simulink model "ACC_RL_new"  (R2022a)
settings: Solver=FixedStepAuto  StartTime=0.0  StopTime=T  FixedStep=Ts  RelTol=1e-3
StartFcn:
  | a_lead_seed = simCount;
  | simCount = simCount + 1;
undefined symbols (not defined in the file): amax_ego, amax_lead, amin_ego, amin_lead, change_freq, D_default, isTerminate, rewardWeights, t_gap, Ts, v0_ego, v0_lead, v_set, x0_ego, x0_lead
libraries: simulink x5, rllib x1
settings Model: Creator=The MathWorks, Inc.  LastModifiedBy=momentumlab
settings SolverCC: AlgebraicLoopSolver=TrustRegion
settings DataIOCC: ReturnWorkspaceOutputs=off
settings DebuggingCC: UnconnectedInputMsg=warning  UnconnectedOutputMsg=warning  UnconnectedLineMsg=warning  SFMachineParentedDataDiag=warning  ArithmeticOperatorsInVariantConditions=warning
settings SFSimCC: SimUseLocalCustomCode=off  CustomCodeUndefinedFunction=UseInterfaceOnly
settings RTWCC: RTWUseLocalCustomCode=off  DLArmComputeVersion=19.05
settings CodeAppCC: StateflowObjectComments=on

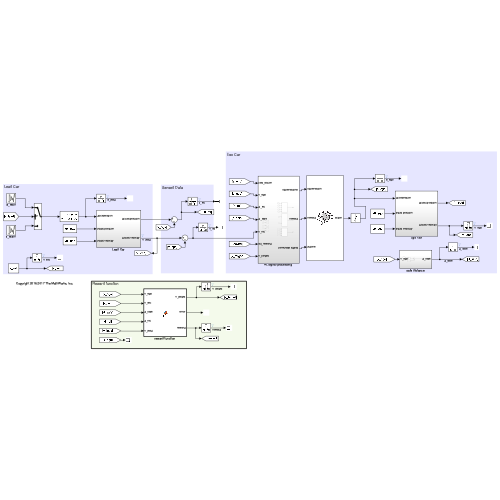
[thumbnail: Simulink's stored preview of the top-level diagram]
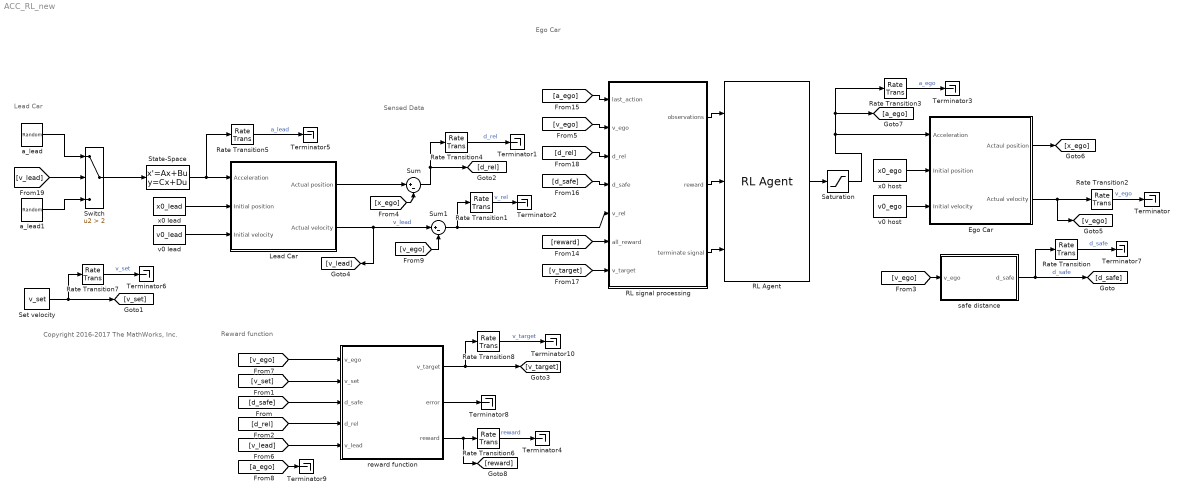
== system ACC_RL_new ==
  note: Reward function
  note: Sensed Data
  note: Lead Car
  note: Ego Car
  note: Copyright 2016-2017 The MathWorks, Inc.
  Ego Car : Subsystem
  Lead Car : Subsystem
  RL Agent : rllib/RL Agent  Agent=agent  ExternalActionAsInput=off  ProvideLastAction=off  ProvideCumRwd=off  TreatAsDirectFeedthrough=on  UseStrictObservationDataTypes=off
  "RL signal processing " : Subsystem
  Rate Transition{,1..8} (9 alike) : RateTransition  OutPortSampleTime=Ts_data
  Saturation : Saturate  UpperLimit=amax_ego  LowerLimit=amin_ego
  Set velocity : Constant  Value=v_set  SampleTime=Ts
  State-Space : StateSpace  A=-10  B=10  D=0  InitialCondition=0
  Sum : Sum  Inputs=|+-
  Sum1 : Sum  Inputs=|+-
  Switch : Switch  Criteria=u2 > Threshold  Threshold=2  SaturateOnIntegerOverflow=off  InputSameDT=off
  Terminator{,1..10} (11 alike) : Terminator
  a_lead : UniformRandomNumber  Minimum=amin_lead  Maximum=amax_lead  Seed=a_lead_seed  SampleTime=change_freq  VectorParams1D=off
  a_lead1 : UniformRandomNumber  Minimum=0  Maximum=amax_lead  Seed=a_lead_seed  SampleTime=change_freq  VectorParams1D=off
  reward function : MATLAB Function  TreatAsAtomicUnit=on
  safe distance : Subsystem
  v0 host : Constant  Value=v0_ego  SampleTime=Ts
  v0 lead : Constant  Value=v0_lead  SampleTime=Ts
  x0 host : Constant  Value=x0_ego  SampleTime=Ts
  x0 lead : Constant  Value=x0_lead  SampleTime=Ts
  wires:
  x0 lead/1 -> Lead Car/2(Initial position)
  v0 lead/1 -> Lead Car/3(Initial velocity)
  x0 host/1 -> Ego Car/2(Initial position)
  v0 host/1 -> Ego Car/3(Initial velocity)
  Lead Car/1(Actual position) -> Sum/1
  Lead Car/2(Actual velocity) -> Sum1/1, [v_lead]  "v_lead"
  Switch/1 -> State-Space/1
  safe distance/1(d_safe) -> Rate Transition/1, [d_safe]  "d_safe"
  Ego Car/2(Actual velocity) -> Rate Transition2/1, [v_ego]
  Saturation/1 -> Ego Car/1(Acceleration), Rate Transition3/1, [a_ego]
  State-Space/1 -> Rate Transition5/1, Lead Car/1(Acceleration)
  [v_set] -> reward function/2(v_set)
  [d_safe] -> reward function/3(d_safe)
  [d_rel] -> reward function/4(d_rel)
  [v_ego] -> safe distance/1(v_ego)
  Ego Car/1(Actaul position) -> [x_ego]
  Sum/1 -> [d_rel], Rate Transition4/1
  Sum1/1 -> "RL signal processing "/5(v_rel), Rate Transition1/1
  [x_ego] -> Sum/2
  reward function/3(reward) -> Rate Transition6/1, [reward]
  [v_ego] -> "RL signal processing "/2(v_ego)
  [v_lead] -> reward function/5(v_lead)
  [v_ego] -> reward function/1(v_ego)
  [v_ego] -> Sum1/2
  Set velocity/1 -> Rate Transition7/1, [v_set]
  RL Agent/1 -> Saturation/1
  "RL signal processing "/1(observations) -> RL Agent/1
  "RL signal processing "/2(reward) -> RL Agent/2
  "RL signal processing "/3(terminate signal) -> RL Agent/3
  [a_ego] -> "RL signal processing "/1(last_action)
  [d_safe] -> "RL signal processing "/4(d_safe)
  [v_target] -> "RL signal processing "/7(v_target)
  [d_rel] -> "RL signal processing "/3(d_rel)
  a_lead/1 -> Switch/1
  [v_lead] -> Switch/2
  a_lead1/1 -> Switch/3
  reward function/2(error) -> Terminator8/1
  [a_ego] -> Terminator9/1
  reward function/1(v_target) -> Rate Transition8/1, [v_target]
  [reward] -> "RL signal processing "/6(all_reward)
  Rate Transition6/1 -> Terminator4/1  "reward"
  Rate Transition7/1 -> Terminator6/1  "v_set"
  Rate Transition5/1 -> Terminator5/1  "a_lead"
  Rate Transition4/1 -> Terminator1/1  "d_rel"
  Rate Transition1/1 -> Terminator2/1  "v_rel"
  Rate Transition3/1 -> Terminator3/1  "a_ego"
  Rate Transition2/1 -> Terminator/1  "v_ego"
  Rate Transition/1 -> Terminator7/1  "d_safe"
  Rate Transition8/1 -> Terminator10/1  "v_target"

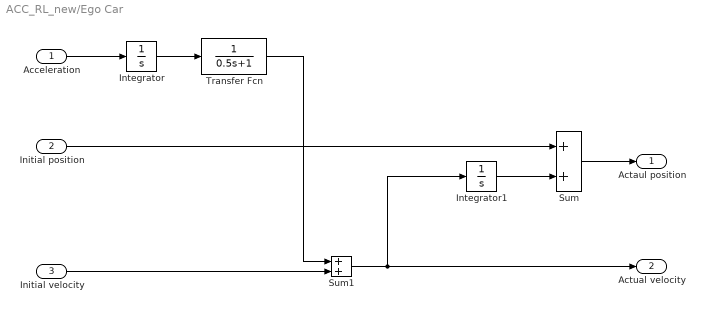
== system ACC_RL_new/Ego Car ==
  Acceleration : Inport
  Initial position : Inport  Port=2
  Initial velocity : Inport  Port=3
  Integrator : Integrator
  Integrator1 : Integrator
  Sum : Sum
  Sum1 : Sum
  Transfer Fcn : TransferFcn  Denominator=[0.5 1]
  Actaul position : Outport  VectorParamsAs1DForOutWhenUnconnected=off
  Actual velocity : Outport  Port=2  VectorParamsAs1DForOutWhenUnconnected=off
  wires:
  Sum1/1 -> Integrator1/1, Actual velocity/1
  Initial velocity/1 -> Sum1/2
  Sum/1 -> Actaul position/1
  Transfer Fcn/1 -> Sum1/1
  Integrator/1 -> Transfer Fcn/1
  Acceleration/1 -> Integrator/1
  Initial position/1 -> Sum/1
  Integrator1/1 -> Sum/2

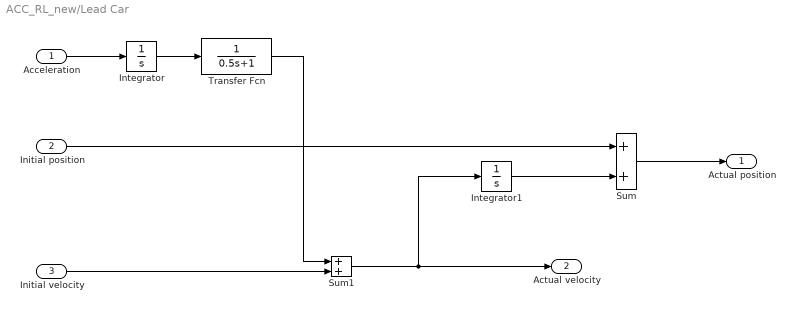
== system ACC_RL_new/Lead Car ==
  Acceleration : Inport
  Initial position : Inport  Port=2
  Initial velocity : Inport  Port=3
  Integrator : Integrator
  Integrator1 : Integrator
  Sum : Sum
  Sum1 : Sum
  Transfer Fcn : TransferFcn  Denominator=[0.5 1]
  Actual position : Outport  VectorParamsAs1DForOutWhenUnconnected=off
  Actual velocity : Outport  Port=2  VectorParamsAs1DForOutWhenUnconnected=off
  wires:
  Transfer Fcn/1 -> Sum1/1
  Initial velocity/1 -> Sum1/2
  Sum/1 -> Actual position/1
  Integrator/1 -> Transfer Fcn/1
  Sum1/1 -> Integrator1/1, Actual velocity/1
  Acceleration/1 -> Integrator/1
  Initial position/1 -> Sum/1
  Integrator1/1 -> Sum/2

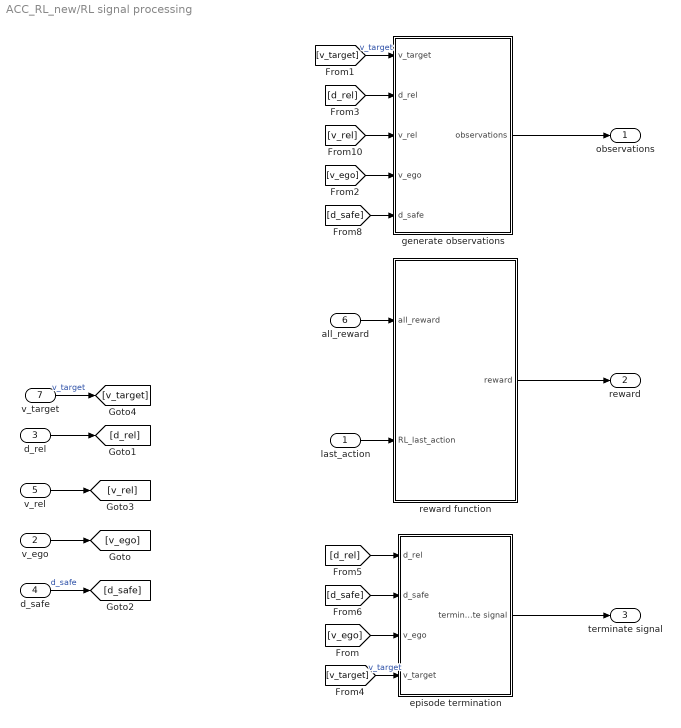
== system ACC_RL_new/RL signal processing  ==
  last_action : Inport
  v_ego : Inport  Port=2
  d_rel : Inport  Port=3
  d_safe : Inport  Port=4
  v_rel : Inport  Port=5
  all_reward : Inport  Port=6
  v_target : Inport  Port=7
  episode termination : Subsystem
  generate observations : Subsystem
  reward function : Subsystem
  observations : Outport
  reward : Outport  Port=2
  terminate signal : Outport  Port=3
  wires:
  last_action/1 -> reward function/2(RL_last_action)
  [v_target] -> generate observations/1(v_target)  "v_target"
  v_ego/1 -> [v_ego]
  d_safe/1 -> [d_safe]  "d_safe"
  generate observations/1(observations) -> observations/1
  reward function/1(reward) -> reward/1
  episode termination/1(terminate signal) -> terminate signal/1
  [v_ego] -> episode termination/3(v_ego)
  [v_ego] -> generate observations/4(v_ego)
  [d_rel] -> generate observations/2(d_rel)
  [d_rel] -> episode termination/1(d_rel)
  [d_safe] -> episode termination/2(d_safe)
  [d_safe] -> generate observations/5(d_safe)
  [v_rel] -> generate observations/3(v_rel)
  d_rel/1 -> [d_rel]
  v_rel/1 -> [v_rel]
  all_reward/1 -> reward function/1(all_reward)
  v_target/1 -> [v_target]  "v_target"
  [v_target] -> episode termination/4(v_target)  "v_target"

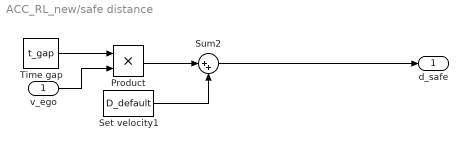
== system ACC_RL_new/safe distance ==
  v_ego : Inport
  Product : Product
  Set velocity1 : Constant  Value=D_default  SampleTime=Ts
  Sum2 : Sum  Inputs=|++
  Time gap : Constant  Value=t_gap  SampleTime=Ts
  d_safe : Outport
  wires:
  Time gap/1 -> Product/1
  Sum2/1 -> d_safe/1
  v_ego/1 -> Product/2
  Product/1 -> Sum2/1
  Set velocity1/1 -> Sum2/2

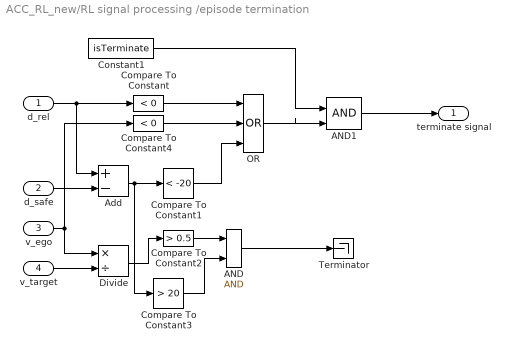
== system ACC_RL_new/RL signal processing /episode termination ==
  d_rel : Inport
  d_safe : Inport  Port=2
  v_ego : Inport  Port=3
  v_target : Inport  Port=4
  AND : Logic  IconShape=distinctive  AllPortsSameDT=off  OutDataTypeStr=boolean
  AND1 : Logic  IconShape=distinctive  AllPortsSameDT=off  OutDataTypeStr=boolean
  Add : Sum  Inputs=+-
  Compare To Constant : simulink/Logic and Bit Operations/Compare To Constant  relop=<  const=0  OutDataTypeStr=boolean
  Compare To Constant1 : simulink/Logic and Bit Operations/Compare To Constant  relop=<  const=-20  OutDataTypeStr=boolean
  Compare To Constant2 : simulink/Logic and Bit Operations/Compare To Constant  relop=>  const=0.5  OutDataTypeStr=boolean
  Compare To Constant3 : simulink/Logic and Bit Operations/Compare To Constant  relop=>  const=20  OutDataTypeStr=boolean
  Compare To Constant4 : simulink/Logic and Bit Operations/Compare To Constant  relop=<  const=0  OutDataTypeStr=boolean
  Constant1 : Constant  Value=isTerminate
  Divide : Product  Inputs=*/
  OR : Logic  Operator=OR  Inputs=3  IconShape=distinctive  AllPortsSameDT=off  OutDataTypeStr=boolean
  Terminator : Terminator
  terminate signal : Outport
  wires:
  d_rel/1 -> Compare To Constant/1, Add/1
  Compare To Constant1/1 -> OR/3
  Add/1 -> Compare To Constant1/1, Compare To Constant3/1
  d_safe/1 -> Add/2
  v_target/1 -> Divide/2
  v_ego/1 -> Compare To Constant4/1, Divide/1
  Divide/1 -> Compare To Constant2/1
  Compare To Constant2/1 -> AND/1
  AND/1 -> Terminator/1
  Compare To Constant3/1 -> AND/2
  Compare To Constant/1 -> OR/1
  Compare To Constant4/1 -> OR/2
  OR/1 -> AND1/2
  AND1/1 -> terminate signal/1
  Constant1/1 -> AND1/1

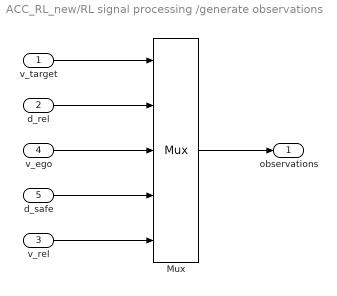
== system ACC_RL_new/RL signal processing /generate observations ==
  v_target : Inport
  d_rel : Inport  Port=2
  v_rel : Inport  Port=3
  v_ego : Inport  Port=4
  d_safe : Inport  Port=5
  Mux : Mux  Inputs=5
  observations : Outport
  wires:
  v_ego/1 -> Mux/3
  v_target/1 -> Mux/1
  Mux/1 -> observations/1
  d_safe/1 -> Mux/4
  v_rel/1 -> Mux/5
  d_rel/1 -> Mux/2

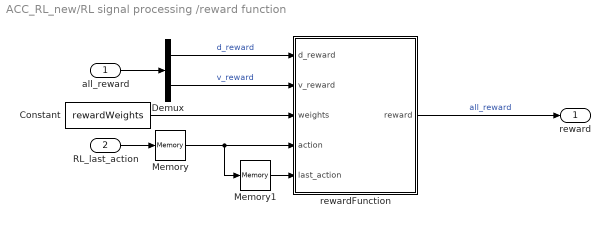
== system ACC_RL_new/RL signal processing /reward function ==
  all_reward : Inport
  RL_last_action : Inport  Port=2
  Constant : Constant  Value=rewardWeights
  Demux : Demux  Outputs=2
  Memory : Memory
  Memory1 : Memory
  rewardFunction : MATLAB Function  TreatAsAtomicUnit=on
  reward : Outport
  wires:
  rewardFunction/1(reward) -> reward/1  "all_reward"
  RL_last_action/1 -> Memory/1
  all_reward/1 -> Demux/1
  Demux/1 -> rewardFunction/1(d_reward)  "d_reward"
  Demux/2 -> rewardFunction/2(v_reward)  "v_reward"
  Constant/1 -> rewardFunction/3(weights)
  Memory/1 -> Memory1/1, rewardFunction/4(action)
  Memory1/1 -> rewardFunction/5(last_action)

== matlab function ACC_RL_new/reward function ==
  data: v_target output; error output; v_ego input; reward output; v_set input; d_safe input; d_rel input; v_lead input
function [v_target, error, reward]= fcn(v_ego, v_set, d_safe, d_rel, v_lead)


% If the relative distance is less than the safe distance, 
% the ego car tracks the minimum of the lead car velocity and driver-set velocity

if d_rel <= d_safe
    v_target = min(v_set, v_lead);
else
    v_target = v_set;
end

v_error = v_ego - v_target;

% reward for velocity [-1,1]
v_reward = -2*tanh(abs(v_error/2)) + 1;

% reward for distance [-1,1]
d_error = d_rel - d_safe;
if d_error >= 0
    d_reward = 1;
else
    d_reward = tanh(d_error/3);
end

% output reward
error = [d_error, v_error];
reward = [d_reward, v_reward];

== matlab function ACC_RL_new/RL signal processing /reward function/rewardFunction ==
  data: d_reward input; reward output; v_reward input; weights input; action input; last_action input
function reward = fcn(d_reward,v_reward,weights, action, last_action)




stable_reward = -2*tanh(abs(action-last_action))+1;

% output reward
% error = [d_error, v_error];
% reward = [d_reward, v_reward];
reward = d_reward*weights(1) + v_reward*weights(2)+stable_reward*weights(3);
